simulink model "sim_01_a_LeftSide"  (R2022a)
settings: Solver=VariableStepAuto  StartTime=0.0  StopTime=25  RelTol=1e-3
settings Model: Creator=Eshmith  LastModifiedBy=Eshmith

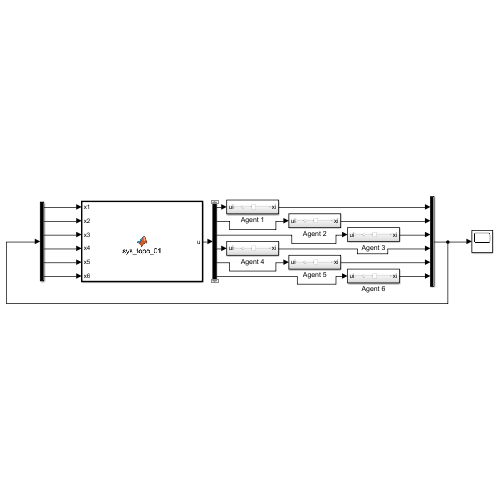
[thumbnail: Simulink's stored preview of the top-level diagram]
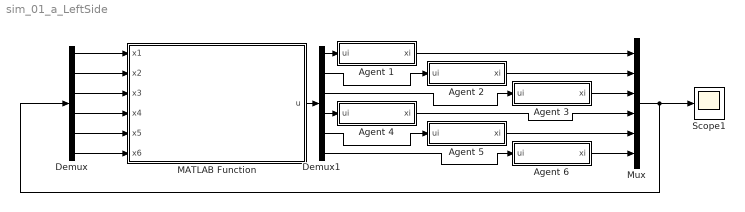
== system sim_01_a_LeftSide ==
  Agent 1 : Subsystem
  Agent 2 : Subsystem
  Agent 3 : Subsystem
  Agent 4 : Subsystem
  Agent 5 : Subsystem
  Agent 6 : Subsystem
  Demux : Demux  Outputs=6
  Demux1 : Demux  Outputs=6
  MATLAB Function : MATLAB Function  TreatAsAtomicUnit=on
  Mux : Mux  Inputs=6
  Scope1 : Scope
  wires:
  Demux1/2 -> Agent 2/1(ui)
  Demux1/4 -> Agent 4/1(ui)
  Demux1/5 -> Agent 5/1(ui)
  Demux1/6 -> Agent 6/1(ui)
  Demux/1 -> MATLAB Function/1(x1)
  Demux/2 -> MATLAB Function/2(x2)
  Demux/3 -> MATLAB Function/3(x3)
  Demux/4 -> MATLAB Function/4(x4)
  Demux/5 -> MATLAB Function/5(x5)
  Demux/6 -> MATLAB Function/6(x6)
  Mux/1 -> Demux/1, Scope1/1
  Agent 1/1(xi) -> Mux/1
  Agent 2/1(xi) -> Mux/2
  Agent 3/1(xi) -> Mux/3
  Agent 4/1(xi) -> Mux/4
  Agent 5/1(xi) -> Mux/5
  Agent 6/1(xi) -> Mux/6
  Demux1/3 -> Agent 3/1(ui)
  MATLAB Function/1(u) -> Demux1/1
  Demux1/1 -> Agent 1/1(ui)

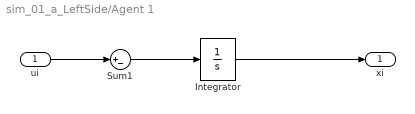
== system sim_01_a_LeftSide/Agent 1 ==
  ui : Inport
  Integrator : Integrator  InitialCondition=10
  Sum1 : Sum  Inputs=|+-
  xi : Outport
  wires:
  Sum1/1 -> Integrator/1
  ui/1 -> Sum1/1
  Integrator/1 -> xi/1

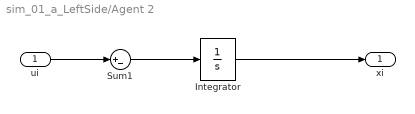
== system sim_01_a_LeftSide/Agent 2 ==
  ui : Inport
  Integrator : Integrator  InitialCondition=1
  Sum1 : Sum  Inputs=|+-
  xi : Outport
  wires:
  Sum1/1 -> Integrator/1
  ui/1 -> Sum1/1
  Integrator/1 -> xi/1

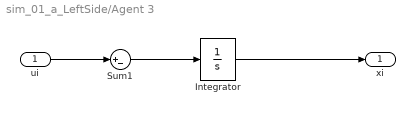
== system sim_01_a_LeftSide/Agent 3 ==
  ui : Inport
  Integrator : Integrator  InitialCondition=2
  Sum1 : Sum  Inputs=|+-
  xi : Outport
  wires:
  Sum1/1 -> Integrator/1
  ui/1 -> Sum1/1
  Integrator/1 -> xi/1

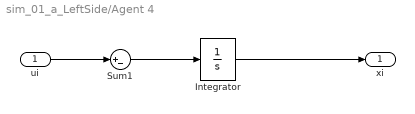
== system sim_01_a_LeftSide/Agent 4 ==
  ui : Inport
  Integrator : Integrator  InitialCondition=3
  Sum1 : Sum  Inputs=|+-
  xi : Outport
  wires:
  Sum1/1 -> Integrator/1
  ui/1 -> Sum1/1
  Integrator/1 -> xi/1

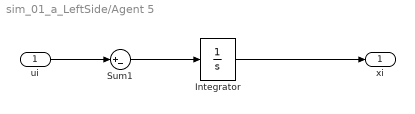
== system sim_01_a_LeftSide/Agent 5 ==
  ui : Inport
  Integrator : Integrator  InitialCondition=4
  Sum1 : Sum  Inputs=|+-
  xi : Outport
  wires:
  Sum1/1 -> Integrator/1
  ui/1 -> Sum1/1
  Integrator/1 -> xi/1

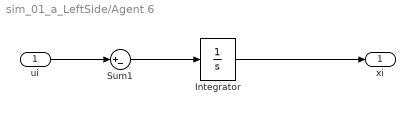
== system sim_01_a_LeftSide/Agent 6 ==
  ui : Inport
  Integrator : Integrator  InitialCondition=5
  Sum1 : Sum  Inputs=|+-
  xi : Outport
  wires:
  Sum1/1 -> Integrator/1
  ui/1 -> Sum1/1
  Integrator/1 -> xi/1

== matlab function sim_01_a_LeftSide/MATLAB Function ==
  data: x1 input; u output; x2 input; x3 input; x4 input; x5 input; x6 input
function u = sys_topo_01(x1, x2, x3, x4, x5, x6)

L = [ 0  0  0  0  0  0;
     -1 +1  0  0  0  0;
      0 -1 +1  0  0  0;
      0  0 -1 +1  0  0;
      0  0 -1 -1 +2  0;
      0  0  0  0 -1 +1;
    ];

states = [x1, x2, x3, x4, x5, x6]';

u = -L*states;

end
